simulink model "Bai5A_1"  (R2015a)
settings: Solver=ode45  StartTime=0.0  StopTime=10.0  RelTol=1e-3
libraries: dspsrcs4 x2, commchan3 x1, commsink2 x1, commutil2 x1, commfilt2 x1, commrandsrc2 x1, dspstat3 x1
settings Model: CovSFcnEnable=off  Creator=Admin  LastModifiedBy=Win 10
settings DebuggingCC: SolverPrmCheckMsg=warning

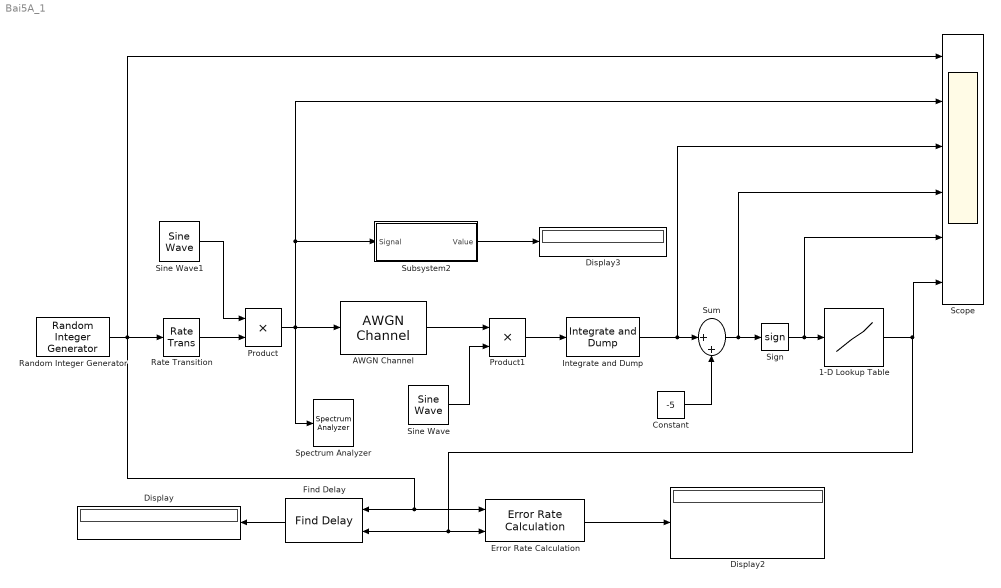
== system Bai5A_1 ==
  1-D Lookup Table : Lookup_n-D  NumberOfTableDimensions=1  BreakpointsForDimension1=[-5:5]  Table=tanh([-5:5])  InternalRulePriority=Speed  RndMeth=Simplest  InputSameDT=on
  AWGN Channel : commchan3/AWGN Channel  InputProcessing=Columns as channels (frame based)  seed=67  noiseMode="Signal to noise ratio  (Eb/No)"  EbNodB=10  EsNodB=10  SNRdB=10  bitsPerSym=1  Ps=1  Tsym=1  variance=1
  Constant : Constant  Value=-5  SampleTime=1/1000
  Display : Display
  Display2 : Display
  Display3 : Display
  Error Rate Calculation : commsink2/Error Rate Calculation  N=0  st_delay=0  cp_mode=Entire frame  subframe=[]  PMode=Port  WsName=ErrorVec  RsMode2=off  stop=off  numErr=100  maxBits=1e6
  Find Delay : commutil2/Find Delay  corrLength=200  chgSigOP=off  stopUpdate=off  numConstDelay=3
  Integrate and Dump : commfilt2/Integrate and Dump  obssamples=8  offsetsamples=0  nodump=off  roundingMode=Floor  overflowMode=off
  Product : Product
  Product1 : Product
  Random Integer Generator : commrandsrc2/Random Integer Generator  mul=2  seed=37  Ts=1/1000  frameBased=off  sampPerFrame=1  orient=on  outDataType=double
  Rate Transition : RateTransition  OutPortSampleTime=1/1000
  Scope : Scope  NumInputPorts=6
      settings: YMin=-5~-5~-5~-5~-5~-5  YMax=5~5~5~5~5~5
  Sign : Signum
  Sine Wave : dspsrcs4/Sine Wave  Amplitude=1  Frequency=100  Phase=0  SampleMode=Discrete  OutComplex=Real  CompMethod=Trigonometric fcn  TableSize=Speed  SampleTime=1/1000  SamplesPerFrame=1  ResetState=Restart at time zero  dataType=double  wordLen=16  udDataType=sfix(16)  fracBitsMode=Best precision  numFracBits=15  OutDataTypeStr=double  LastOutDataTypeStr=double
  Sine Wave1 : dspsrcs4/Sine Wave  Amplitude=1  Frequency=100  Phase=0  SampleMode=Discrete  OutComplex=Real  CompMethod=Trigonometric fcn  TableSize=Speed  SampleTime=1/1000  SamplesPerFrame=1  ResetState=Restart at time zero  dataType=double  wordLen=16  udDataType=sfix(16)  fracBitsMode=Best precision  numFracBits=15  OutDataTypeStr=double  LastOutDataTypeStr=double
  Spectrum Analyzer : SpectrumAnalyzer
  Subsystem2 : Subsystem
  Sum : Sum  Inputs=|++
  wires:
  Random Integer Generator/1 -> Error Rate Calculation/1, Find Delay/1, Scope/1, Rate Transition/1
  Rate Transition/1 -> Product/2
  Sine Wave1/1 -> Product/1
  Product/1 -> Spectrum Analyzer/1, Subsystem2/1(Signal), Scope/2, AWGN Channel/1
  AWGN Channel/1 -> Product1/1
  Sine Wave/1 -> Product1/2
  Find Delay/1 -> Display/1
  Subsystem2/1(Value) -> Display3/1
  Error Rate Calculation/1 -> Display2/1
  Constant/1 -> Sum/2
  Sum/1 -> Scope/4, Sign/1
  Sign/1 -> Scope/5, 1-D Lookup Table/1
  Product1/1 -> Integrate and Dump/1
  Integrate and Dump/1 -> Scope/3, Sum/1
  1-D Lookup Table/1 -> Error Rate Calculation/2, Find Delay/2, Scope/6

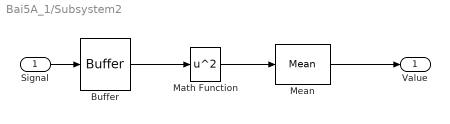
== system Bai5A_1/Subsystem2 ==
  Signal : Inport
  Buffer : Buffer  TreatMby1Signals=One channel
  Math Function : Math  Operator=square  SaturateOnIntegerOverflow=on
  Mean : dspstat3/Mean  run=off  reset_popup=None  InputProcessing=Columns as channels (frame based)  directionMode=Each column  dimension=1  treatSBRowAsCol=off  roiEnable=off  roiType=Rectangles  roiPortion=Entire ROI  roiOutput=Individual statistics for each ROI  roiFlag=off  outputDataTypeStr=Inherit: Same as accumulator  outputLastDataTypeStr=Inherit: Same as accumulator  outputMin=[]  outputMax=[]  roundingMode=Floor  overflowMode=off
  Value : Outport
  wires:
  Math Function/1 -> Mean/1
  Mean/1 -> Value/1
  Buffer/1 -> Math Function/1
  Signal/1 -> Buffer/1
